simulink model "neurocircle"  (Simulink 8.3)
settings: Solver=ode3  StartTime=0.0  StopTime=1500  FixedStep=0.3  MinStep=0.01  RelTol=1e-3
libraries: simulink x3
settings Model: Creator=Administrator  LastModifiedBy=jackyjing
settings OptimizationCC: ExpressionDepthLimit=2147483647
settings DebuggingCC: FcnCallInpInsideContextMsg=UseLocalSettings

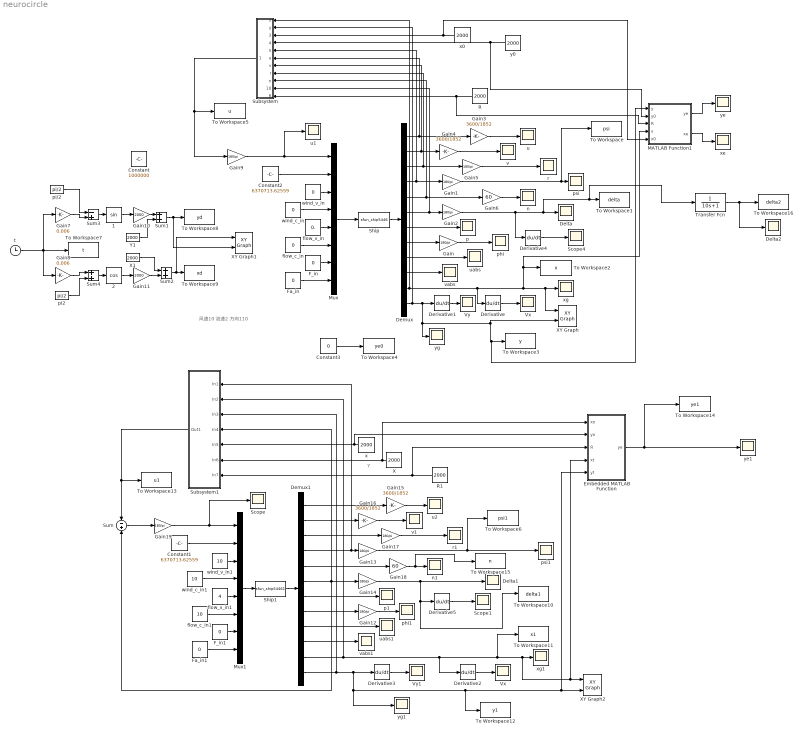
== system neurocircle ==
  note: 风速10 流速2 方向110
  note: Y
  "  1" : Trigonometry
  " 2" : Trigonometry  Operator=cos
  Constant : Constant  Value=1000000
  Constant1 : Constant  Value=6370713.62559
  Constant2 : Constant  Value=6370713.62559
  Constant3 : Constant  Value=0
  Delta : Scope
      settings: TickLabels=on  TimeRange=1500  YMin=-20  YMax=17.5  SaveName=ScopeData5
  Delta1 : Scope
      settings: TickLabels=on  TimeRange=1500  YMin=-17.5  YMax=20  SaveName=ScopeData31
  Delta2 : Scope
      settings: TickLabels=on  TimeRange=1500  YMin=-22.5  YMax=22.5  SaveName=ScopeData48
  Demux : Demux  Outputs=12
  Demux1 : Demux  Outputs=12
  Derivative{,1..5} (6 alike) : Derivative
  Embedded MATLAB Function : MATLAB Function  TreatAsAtomicUnit=on
  F_in : Constant  Value=0
  F_in1 : Constant  Value=0
  Fa_in : Constant  Value=0
  Fa_in1 : Constant  Value=0
  Gain{,1..2,5,9,12..14,17,19} (10 alike) : Gain  Gain=180/pi
  Gain10 : Gain  Gain=2000
  Gain11 : Gain  Gain=2000
  Gain{3..4,15..16} (4 alike) : Gain  Gain=3600/1852
  Gain18 : Gain  Gain=60
  Gain6 : Gain  Gain=60
  Gain7 : Gain  Gain=0.006
  Gain8 : Gain  Gain=0.006
  MATLAB Function1 : MATLAB Function  TreatAsAtomicUnit=on
  Mux : Mux  Inputs=8
  Mux1 : Mux  Inputs=8
  R : Constant  Value=2000
  R1 : Constant  Value=2000
  Scope : Scope
      settings: TimeRange=1000  YMin=-0.6  YMax=0.8  SaveName=ScopeData32
  Scope1 : Scope
      settings: YMin=-0.005  YMax=0.002  SaveName=ScopeData33
  Scope4 : Scope
      settings: YMin=-0.005  YMax=0.002  SaveName=ScopeData18
  Ship : S-Function  FunctionName=sfun_ship5446  EnableBusSupport=off
  Ship1 : S-Function  FunctionName=sfun_ship54461  EnableBusSupport=off
  Subsystem : Subsystem
  Subsystem1 : Subsystem
  Sum : Sum  Inputs=-|+
  Sum1 : Sum
  Sum2 : Sum
  Sum3 : Sum  Inputs=-+
  Sum4 : Sum
  To Workspace : ToWorkspace  VariableName=psi  SampleTime=-1
  To Workspace1 : ToWorkspace  VariableName=delta  SampleTime=-1
  To Workspace10 : ToWorkspace  VariableName=delta1  SampleTime=-1
  To Workspace11 : ToWorkspace  VariableName=x1  SampleTime=-1
  To Workspace12 : ToWorkspace  VariableName=y1  SampleTime=-1
  To Workspace13 : ToWorkspace  VariableName=u1  SampleTime=-1
  To Workspace14 : ToWorkspace  VariableName=ye1  SampleTime=-1
  To Workspace15 : ToWorkspace  VariableName=n  SampleTime=-1
  To Workspace16 : ToWorkspace  VariableName=delta2  SampleTime=-1
  To Workspace2 : ToWorkspace  VariableName=x  SampleTime=-1
  To Workspace3 : ToWorkspace  VariableName=y  SampleTime=-1
  To Workspace4 : ToWorkspace  VariableName=ye0  SampleTime=-1
  To Workspace5 : ToWorkspace  VariableName=u  SampleTime=-1
  To Workspace6 : ToWorkspace  VariableName=psi1  SampleTime=-1
  To Workspace7 : ToWorkspace  VariableName=t  SampleTime=-1
  To Workspace8 : ToWorkspace  VariableName=yd  SampleTime=-1
  To Workspace9 : ToWorkspace  VariableName=xd  SampleTime=-1
  Transfer Fcn : TransferFcn  Denominator=[10 1]
  Vx : Scope
      settings: TickLabels=on  SaveName=ScopeData8
  "Vx " : Scope
      settings: TickLabels=on  SaveName=ScopeData34
  Vy : Scope
      settings: TickLabels=on  SaveName=ScopeData9
  Vy1 : Scope
      settings: TickLabels=on  SaveName=ScopeData35
  X : Constant  Value=2000
  X1 : Constant  Value=2000
  XY Graph : simulink/Sinks/XY Graph  xmin=-1000  xmax=5000  ymin=-1000  ymax=5000  st=-1
  XY Graph1 : simulink/Sinks/XY Graph  xmin=-1000  xmax=5000  ymin=-1000  ymax=5000  st=-1
  XY Graph2 : simulink/Sinks/XY Graph  xmin=-1500  xmax=5000  ymin=-1500  ymax=5000  st=-1
  Y1 : Constant  Value=2000
  flow_c_in : Constant  Value=0
  flow_c_in1 : Constant  Value=10
  flow_v_in : Constant  Value=0.
  flow_v_in1 : Constant  Value=4
  n : Scope
      settings: TickLabels=on  YMin=38.5  YMax=46.5  SaveName=ScopeData4
  n1 : Scope
      settings: TickLabels=on  YMin=38.5  YMax=46.5  SaveName=ScopeData36
  p : Scope
      settings: TickLabels=on  SaveName=ScopeData10
  p1 : Scope
      settings: TickLabels=on  SaveName=ScopeData37
  phi : Scope
      settings: YMin=-0.00175  YMax=0.0015  SaveName=ScopeData11
  phi1 : Scope
      settings: YMin=-0.00175  YMax=0.0015  SaveName=ScopeData38
  pi/2 : Constant  Value=pi/2
  "pi2   " : Constant  Value=pi/2
  psi : Scope
      settings: TickLabels=on  TimeRange=44.44444444444434  YMin=52  YMax=60.5  SaveName=ScopeData3
  psi1 : Scope
      settings: TickLabels=on  TimeRange=500  YMin=9.9825  YMax=10.01  SaveName=ScopeData39
  r : Scope
      settings: TickLabels=on  SaveName=ScopeData2
  r1 : Scope
      settings: TickLabels=on  SaveName=ScopeData40
  t : Clock
  u : Scope
      settings: TickLabels=on  YMin=28.45  YMax=29.45
  u1 : Scope
      settings: TickLabels=on  TimeRange=1500  YMin=-35000  YMax=35000  SaveName=ScopeData15
  u2 : Scope
      settings: TickLabels=on  TimeRange=1500  YMin=10  YMax=30  SaveName=ScopeData41
  uabs : Scope
      settings: TickLabels=on  YMin=10.75  YMax=15  SaveName=ScopeData6
  uabs1 : Scope
      settings: TickLabels=on  YMin=10.75  YMax=15  SaveName=ScopeData42
  v : Scope
      settings: TickLabels=on
  v1 : Scope
      settings: TickLabels=on  YMin=-0.3  YMax=0.15  SaveName=ScopeData43
  vabs : Scope
      settings: TickLabels=on  YMin=-1.75  YMax=0  SaveName=ScopeData7
  vabs1 : Scope
      settings: TickLabels=on  YMin=-1.75  YMax=0  SaveName=ScopeData44
  wind_c_in : Constant  Value=0
  wind_c_in1 : Constant  Value=10
  wind_v_in : Constant  Value=0
  wind_v_in1 : Constant  Value=10
  x : Constant  Value=2000
  x0 : Constant  Value=2000
  xe : Scope
      settings: TickLabels=on  YMin=-475  YMax=50  SaveName=ScopeData16
  xg : Scope
      settings: TickLabels=on  YMin=250  YMax=475  SaveName=ScopeData12
  xg1 : Scope
      settings: TickLabels=on  YMin=-100  YMax=1100  SaveName=ScopeData45
  y0 : Constant  Value=2000
  ye : Scope
      settings: TickLabels=on  YMin=-550  YMax=250  SaveName=ScopeData17
  ye1 : Scope
      settings: TickLabels=on  YMin=-100  YMax=850  SaveName=ScopeData47
  yg : Scope
      settings: TickLabels=on  YMin=250  YMax=475  SaveName=ScopeData13
  yg1 : Scope
      settings: TickLabels=on  YMin=-800  YMax=600  SaveName=ScopeData46
  wires:
  Ship/1 -> Demux/1
  Demux/1 -> Subsystem/6(u), Gain3/1
  Demux/2 -> Subsystem/7(v), Gain4/1
  Demux/3 -> Subsystem/8(r), Gain5/1
  Demux/5 -> Subsystem/9(n), Gain6/1
  Demux/7 -> p/1
  Demux/8 -> Gain/1
  Demux/4 -> Gain1/1, Subsystem/5(psi)
  Gain/1 -> phi/1
  Gain3/1 -> u/1
  Gain4/1 -> v/1
  Gain5/1 -> r/1
  Gain6/1 -> n/1
  Demux/9 -> uabs/1
  Demux/10 -> vabs/1
  Demux/12 -> Subsystem/2(y), Derivative1/1, yg/1, MATLAB Function1/1(y), To Workspace3/1, XY Graph/2
  Demux/11 -> Subsystem/1(x), Derivative/1, XY Graph/1, xg/1, MATLAB Function1/4(x), To Workspace2/1
  Derivative/1 -> Vx/1
  Derivative1/1 -> Vy/1
  wind_v_in/1 -> Mux/3
  wind_c_in/1 -> Mux/4
  flow_v_in/1 -> Mux/5
  F_in/1 -> Mux/7
  Fa_in/1 -> Mux/8
  flow_c_in/1 -> Mux/6
  Mux/1 -> Ship/1
  Constant2/1 -> Mux/2
  Derivative4/1 -> Scope4/1
  Gain9/1 -> u1/1, Mux/1
  y0/1 -> MATLAB Function1/2(y0), Subsystem/4(y0)
  R/1 -> MATLAB Function1/3(R), Subsystem/11(R)
  Sum1/1 -> XY Graph1/2, To Workspace8/1
  "  1"/1 -> Gain10/1
  " 2"/1 -> Gain11/1
  t/1 -> To Workspace7/1, Gain8/1, Gain7/1
  Gain10/1 -> Sum1/1
  Gain11/1 -> Sum2/2
  X1/1 -> Sum2/1
  Y1/1 -> Sum1/2
  Sum3/1 -> "  1"/1
  Gain7/1 -> Sum3/2
  pi/2/1 -> Sum3/1
  Sum4/1 -> " 2"/1
  Gain8/1 -> Sum4/1
  "pi2   "/1 -> Sum4/2
  Demux/6 -> Subsystem/10(Delta), Gain2/1
  Subsystem/1("psi ") -> To Workspace5/1, Gain9/1
  MATLAB Function1/2(xe) -> xe/1
  MATLAB Function1/1(ye) -> ye/1
  x0/1 -> MATLAB Function1/5(x0), Subsystem/3(x0)
  Gain1/1 -> psi/1, To Workspace/1
  Sum2/1 -> XY Graph1/1, To Workspace9/1
  Ship1/1 -> Demux1/1
  Demux1/1 -> Gain15/1
  Demux1/2 -> Gain16/1
  Demux1/3 -> Gain17/1
  Demux1/5 -> Gain18/1
  Demux1/7 -> p1/1
  Demux1/8 -> Gain12/1
  Gain13/1 -> psi1/1, To Workspace6/1
  Gain12/1 -> phi1/1
  Gain15/1 -> u2/1
  Gain16/1 -> v1/1
  Gain17/1 -> r1/1
  Gain18/1 -> To Workspace15/1, n1/1
  Demux1/9 -> uabs1/1
  Demux1/10 -> vabs1/1
  Demux1/12 -> Derivative3/1, yg1/1, To Workspace12/1, Embedded MATLAB Function/5(yt), XY Graph2/2, Subsystem1/3(In3)
  Demux1/11 -> Derivative2/1, To Workspace11/1, Embedded MATLAB Function/4(xt), XY Graph2/1, xg1/1, Subsystem1/2(In2)
  Derivative2/1 -> "Vx "/1
  Derivative3/1 -> Vy1/1
  wind_v_in1/1 -> Mux1/3
  wind_c_in1/1 -> Mux1/4
  flow_v_in1/1 -> Mux1/5
  F_in1/1 -> Mux1/7
  Fa_in1/1 -> Mux1/8
  flow_c_in1/1 -> Mux1/6
  Mux1/1 -> Ship1/1
  Constant1/1 -> Mux1/2
  Sum/1 -> Gain19/1
  Derivative5/1 -> Scope1/1
  Subsystem1/1(Out1) -> Sum/1, To Workspace13/1
  Demux1/4 -> Gain13/1, Subsystem1/1(In1)
  Gain19/1 -> Mux1/1, Scope/1
  x/1 -> Subsystem1/5(In5), Embedded MATLAB Function/2(yo)
  X/1 -> Subsystem1/6(In6), Embedded MATLAB Function/1(xo)
  R1/1 -> Subsystem1/7(In7), Embedded MATLAB Function/3(R)
  Demux1/6 -> Sum/2, Gain14/1, Subsystem1/4(In4)
  Gain14/1 -> To Workspace10/1, Derivative5/1, Delta1/1
  Embedded MATLAB Function/1(ye) -> ye1/1, To Workspace14/1
  Constant3/1 -> To Workspace4/1
  Gain2/1 -> Derivative4/1, Delta/1, Transfer Fcn/1, To Workspace1/1
  Transfer Fcn/1 -> Delta2/1, To Workspace16/1

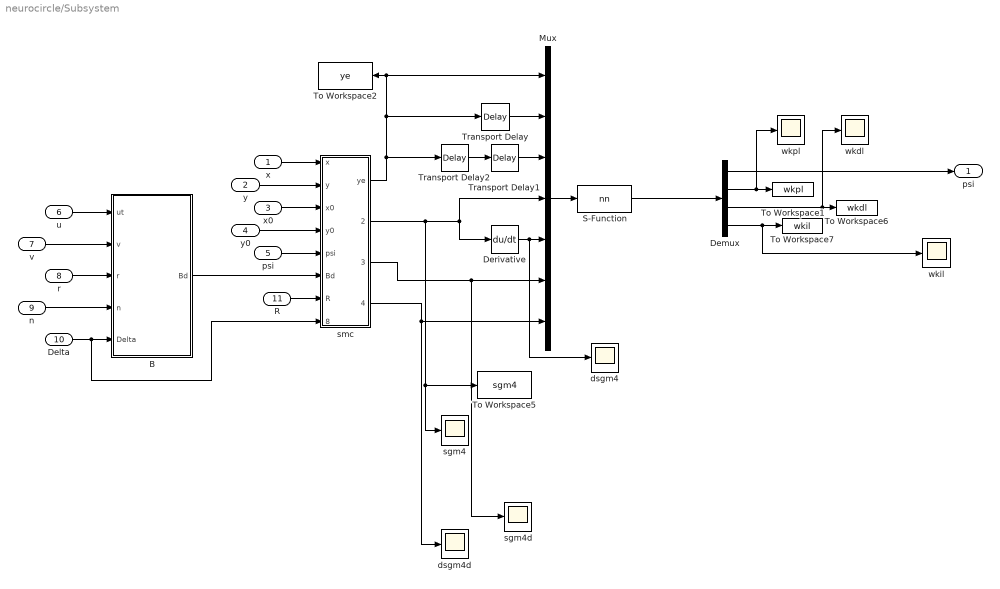
== system neurocircle/Subsystem ==
  x : Inport
  y : Inport  Port=2
  x0 : Inport  Port=3
  y0 : Inport  Port=4
  psi : Inport  Port=5
  u : Inport  Port=6
  v : Inport  Port=7
  r : Inport  Port=8
  n : Inport  Port=9
  Delta : Inport  Port=10
  R : Inport  Port=11
  B : MATLAB Function  TreatAsAtomicUnit=on
  Demux : Demux
  Derivative : Derivative
  Mux : Mux  Inputs=7
  S-Function : S-Function  FunctionName=nn  EnableBusSupport=off
  To Workspace1 : ToWorkspace  VariableName=wkpl  SampleTime=-1
  To Workspace2 : ToWorkspace  VariableName=ye  SampleTime=-1
  To Workspace5 : ToWorkspace  VariableName=sgm4  SampleTime=-1
  To Workspace6 : ToWorkspace  VariableName=wkdl  SampleTime=-1
  To Workspace7 : ToWorkspace  VariableName=wkil  SampleTime=-1
  Transport Delay : TransportDelay  DelayTime=2
  Transport Delay1 : TransportDelay
  Transport Delay2 : TransportDelay
  dsgm4 : Scope
      settings: TickLabels=on  TimeRange=1500  YMin=-4.20046e+11  YMax=-3.80042e+11  SaveName=ScopeData25
  dsgm4d : Scope
      settings: TickLabels=on  TimeRange=1500  YMin=0.00019  YMax=0.00028  SaveName=ScopeData23
  sgm4 : Scope
      settings: TickLabels=on  TimeRange=1500  YMin=-0.00045  YMax=0.0006  SaveName=ScopeData24
  sgm4d : Scope
      settings: TickLabels=on  TimeRange=1500  YMin=0.00975  YMax=0.014  SaveName=ScopeData21
  "smc " : Subsystem
  wkdl : Scope
      settings: TickLabels=on  TimeRange=1500  YMin=0.3  YMax=1  SaveName=ScopeData19
  wkil : Scope
      settings: TickLabels=on  TimeRange=1500  YMin=-0.025  YMax=0.35  SaveName=ScopeData20
  wkpl : Scope
      settings: TickLabels=on  TimeRange=1500  YMin=-0.45  YMax=0.5  SaveName=ScopeData22
  "psi " : Outport
  wires:
  x/1 -> "smc "/1(x)
  y/1 -> "smc "/2(y)
  x0/1 -> "smc "/3(x0)
  y0/1 -> "smc "/4(y0)
  psi/1 -> "smc "/5("psi ")
  u/1 -> B/1(ut)
  v/1 -> B/2(v)
  r/1 -> B/3(r)
  n/1 -> B/4(n)
  Mux/1 -> S-Function/1
  Transport Delay/1 -> Mux/2
  Transport Delay1/1 -> Mux/3
  Derivative/1 -> dsgm4/1, Mux/5
  B/1(Bd) -> "smc "/6(Bd)
  Transport Delay2/1 -> Transport Delay1/1
  R/1 -> "smc "/7(R)
  Delta/1 -> "smc "/8(delta), B/5(Delta)
  S-Function/1 -> Demux/1
  Demux/2 -> To Workspace1/1, wkpl/1
  Demux/3 -> To Workspace6/1, wkdl/1
  Demux/4 -> wkil/1, To Workspace7/1
  Demux/1 -> "psi "/1
  "smc "/1(ye) -> Transport Delay2/1, Transport Delay/1, Mux/1, To Workspace2/1
  "smc "/2(sgm4) -> Mux/4, Derivative/1, To Workspace5/1, sgm4/1
  "smc "/3(sgm4d) -> sgm4d/1, Mux/6
  "smc "/4(dsgm4d) -> Mux/7, dsgm4d/1

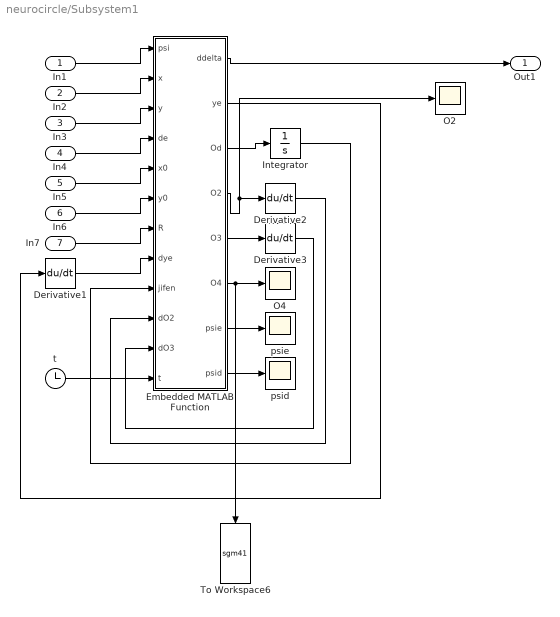
== system neurocircle/Subsystem1 ==
  In1 : Inport
  In2 : Inport  Port=2
  In3 : Inport  Port=3
  In4 : Inport  Port=4
  In5 : Inport  Port=5
  In6 : Inport  Port=6
  In7 : Inport  Port=7
  Derivative1 : Derivative
  Derivative2 : Derivative
  Derivative3 : Derivative
  Embedded MATLAB Function : MATLAB Function  TreatAsAtomicUnit=on
  Integrator : Integrator
  O2 : Scope
      settings: TickLabels=on  TimeRange=500  YMin=-4.5  YMax=3.5  SaveName=ScopeData19
  O4 : Scope
      settings: TickLabels=on  TimeRange=500  YMin=-0.00115  YMax=-0.0001  SaveName=ScopeData18
  To Workspace6 : ToWorkspace  VariableName=sgm41  SampleTime=-1
  psid : Scope
      settings: TickLabels=on  TimeRange=2000  YMin=-2  SaveName=ScopeData20
  psie : Scope
      settings: TickLabels=on  TimeRange=2000  YMin=0.1  YMax=0.8  SaveName=ScopeData17
  t : Clock
  Out1 : Outport
  wires:
  Embedded MATLAB Function/5(O3) -> Derivative3/1
  Derivative3/1 -> Embedded MATLAB Function/11(dO3)
  Embedded MATLAB Function/4(O2) -> O2/1, Derivative2/1
  Derivative2/1 -> Embedded MATLAB Function/10(dO2)
  Integrator/1 -> Embedded MATLAB Function/9(jifen)
  Embedded MATLAB Function/1(ddelta) -> Out1/1
  Embedded MATLAB Function/3(Od) -> Integrator/1
  In1/1 -> Embedded MATLAB Function/1(psi)
  In2/1 -> Embedded MATLAB Function/2(x)
  In3/1 -> Embedded MATLAB Function/3(y)
  Derivative1/1 -> Embedded MATLAB Function/8(dye)
  Embedded MATLAB Function/2(ye) -> Derivative1/1
  In4/1 -> Embedded MATLAB Function/4(de)
  In5/1 -> Embedded MATLAB Function/5(x0)
  In6/1 -> Embedded MATLAB Function/6(y0)
  In7/1 -> Embedded MATLAB Function/7(R)
  Embedded MATLAB Function/7(psie) -> psie/1
  Embedded MATLAB Function/6(O4) -> O4/1, To Workspace6/1
  Embedded MATLAB Function/8(psid) -> psid/1
  t/1 -> Embedded MATLAB Function/12(t)

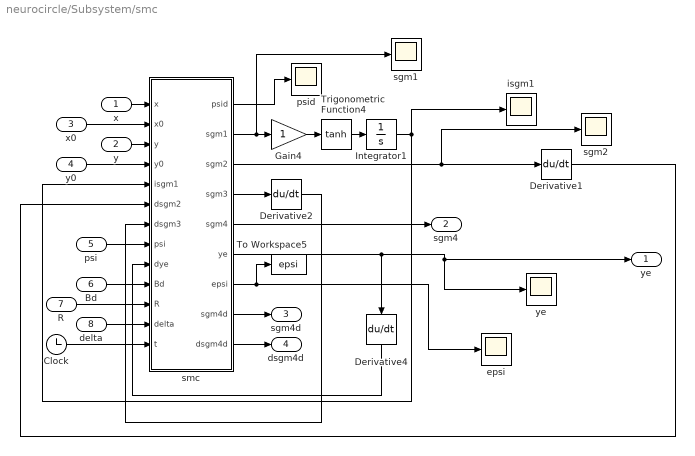
== system neurocircle/Subsystem/smc  ==
  x : Inport
  y : Inport  Port=2
  x0 : Inport  Port=3
  y0 : Inport  Port=4
  "psi " : Inport  Port=5
  Bd : Inport  Port=6
  R : Inport  Port=7
  delta : Inport  Port=8
  Clock : Clock
  Derivative1 : Derivative
  Derivative2 : Derivative
  Derivative4 : Derivative
  Gain4 : Gain
  Integrator1 : Integrator
  To Workspace5 : ToWorkspace  VariableName=epsi  SampleTime=-1
  Trigonometric Function4 : Trigonometry  Operator=tanh
  epsi : Scope
      settings: TickLabels=on  TimeRange=1500  YMin=-0.1  YMax=0.8  SaveName=ScopeData29
  isgm1 : Scope
      settings: TickLabels=on  TimeRange=1500  YMin=-150  YMax=650  SaveName=ScopeData28
  psid : Scope
      settings: TickLabels=on  TimeRange=1500  YMin=-3.5  YMax=3.5  SaveName=ScopeData30
  sgm1 : Scope
      settings: TickLabels=on  TimeRange=1500  YMin=-15  YMax=15  SaveName=ScopeData26
  sgm2 : Scope
      settings: TickLabels=on  TimeRange=1500  YMax=7  SaveName=ScopeData27
  "smc " : MATLAB Function  TreatAsAtomicUnit=on
  "ye " : Scope
      settings: TimeRange=1500  YMin=-700  YMax=900  SaveName=ScopeData14
  ye : Outport
  sgm4 : Outport  Port=2
  sgm4d : Outport  Port=3
  dsgm4d : Outport  Port=4
  wires:
  "smc "/2(sgm1) -> sgm1/1, Gain4/1
  Derivative2/1 -> "smc "/7(dsgm3)
  "smc "/4(sgm3) -> Derivative2/1
  Trigonometric Function4/1 -> Integrator1/1
  Derivative1/1 -> "smc "/6(dsgm2)
  Integrator1/1 -> isgm1/1, "smc "/5(isgm1)
  x/1 -> "smc "/1(x)
  y/1 -> "smc "/3(y)
  x0/1 -> "smc "/2(x0)
  y0/1 -> "smc "/4(y0)
  "smc "/5(sgm4) -> sgm4/1
  "smc "/6(ye) -> "ye "/1, ye/1, Derivative4/1
  Bd/1 -> "smc "/10(Bd)
  Derivative4/1 -> "smc "/9(dye)
  "smc "/8(sgm4d) -> sgm4d/1
  "smc "/9(dsgm4d) -> dsgm4d/1
  R/1 -> "smc "/11(R)
  delta/1 -> "smc "/12(delta)
  "smc "/7(epsi) -> To Workspace5/1, epsi/1
  Gain4/1 -> Trigonometric Function4/1
  "smc "/1(psid) -> psid/1
  "psi "/1 -> "smc "/8(psi)
  "smc "/3(sgm2) -> Derivative1/1, sgm2/1
  Clock/1 -> "smc "/13(t)

== matlab function Subsystem/smc /smc  ==
  data: psid output double; x input double; x0 input double; y input double; y0 input double; isgm1 input double; dsgm2 input double; dsgm3 input double; sgm1 output double; sgm2 output double; sgm3 output double; psi input double; dye input double; sgm4 output double; ye output double; epsi output double; Bd input double; sgm4d output double; dsgm4d output double; R input double; delta input double; t input double
function [psid,sgm1,sgm2,sgm3,sgm4,ye,epsi,sgm4d,dsgm4d]= fcn(x,x0,y,y0,isgm1,dsgm2,dsgm3,psi,dye,Bd,R,delta,t)
%#codegen
% k0=0.8;k1=3;k2=0.0000001;k3=0.0000002;k4=0.04;
%k0=0.8;k1=0.001;k2=0.0000001;k3=0.0000002;k4=0.04;
k0=0.8;k1=4;k2=0.0000001;k3=0.0000001;k4=0.03;
 ye=sqrt((x-x0)^2+(y-y0)^2)-R;
if(atan2((y-y0),(x-x0))<0&&t>700)
    epsi=psi-atan2((y-y0),(x-x0))-pi/2-2*pi;
elseif(atan2((y-y0),(x-x0))>0&&t>1000)
    epsi=psi-atan2((y-y0),(x-x0))-pi/2-2*pi;
else
    epsi=psi-atan2((y-y0),(x-x0))-pi/2;     
end

  psid=atan2((y-y0),(x-x0));
% if(t<=784.2)
%   epsi=psi-psid-pi/2;
% else
%   epsi=0.0473;
% end
% epsi=psi-psid-pi/2;
sgm1=k1*tanh(k0*ye)+dye;
sgm2=epsi+k2*isgm1;
sgm3=k3*tanh(sgm2)+dsgm2;
sgm4=k4*tanh(sgm3)+dsgm3;

sgm4d=Bd; 
dsgm4d=(k4*(sech(sgm3)^2)+k3*(sech(sgm2)^2))*Bd;

== matlab function Subsystem/B ==
  data: ut input double; Bd output double; v input double; r input double; n input double; Delta input double
function Bd  = fcn(ut,v,r,n,Delta)
% function ud = fcn(ut,v,r,n,Delta,phi,dr,sgm4)
V=sqrt(ut*ut+v*v);%u=x(1) v=x(2)

da=10.5;%9.34+0.25;%尾吃水13.8;%12.5;%
df=7.5;%4.97+0.25;%首吃水14.3;%13.8;%
Dh=9.0;%舵高s   ;%11.411.4;;%+7.00+0.25
pa=1.205;%%%**空气密度
Lpp=267.0;%船长
B=39.8;%船宽
Db=6.466;%舵宽
P=9.657;%da螺距
luow=1026;%小luow是密度 水密度
Dp=9.2;%螺旋桨直径
Ds=23.6;%型深
d=(da+df)/2;%吃水
m=(165.89*d*d + 4383.9*d)*1000;%排水量
Cb=m/(Lpp*B*d*1.025*1000);
AR=(d-7.41)/(12.5-7.41)*(81.44-43.14)+43.14;%舵叶面积
d_B=d/B;L_B=Lpp/B;
mx=m/100*(0.398+11.97*Cb*(1+3.73*d_B)-2.89*Cb*L_B*(1+1.13*d_B)+0.175*Cb*L_B*L_B*(1+0.541*d_B)-1.107*L_B*d_B);
my=m*(0.882-0.54*Cb*(1-1.6*d_B)-0.156*L_B*(1-0.673*Cb)+0.826*d_B*L_B*(1-0.678*d_B)-0.638*Cb*d_B*L_B*(1-0.669*d_B));
wp0=0.5*Cb-0.05;
fa=6.13*Dh/Db/(2.25+Dh/Db);
gma=-22.2*(Cb*B/Lpp)*(Cb*B/Lpp)+0.02*(Cb*B/Lpp)+0.68;
gmaR=1.1633-1.98828*Cb+1.3902*Cb*Cb;
tR=0.7382-0.0539*Cb+0.1755*Cb*Cb;
ifaH=0.6784-1.3374*Cb+1.8891*Cb*Cb;
xH=-(0.4+0.1*Cb)*Lpp;
xR=-0.5*Lpp;
xb=1.87;
Jzz=1/100.0*(33-76.85*Cb*(1-0.784*Cb)+3.43*L_B*(1-0.63*Cb))*Lpp*Lpp;
Izz=(1.0+(Cb^4.5))*m*(Lpp*Lpp+power(B,2.4))/24.0;

m33=Izz+Jzz;

beta=atan2((-v),(ut));%u=x(1) v=x(2)
betap=beta+0.5*r*Lpp/V;%r=x(3)
betaR=beta+r*Lpp/V;
wp=wp0*exp(-4.0*betap*betap);
up=(1.0-wp)*ut;%u=x(1)
s=1.0-up/n/P;% n=x(5)
eta=Dp/Dh;

k=0.6;
Gs=eta*k*(2.0-(2.0-k)*s)*s/(1.0-s)/(1.0-s);
s0=1-(1-wp0)*ut/n/P;% n=x(5)u=x(1)
delt0=-s0/57.3;

if(Delta<0)
    K=1.065;
else
    K=0.935;
end
%
uR=up*(1+K*Gs)^0.5;
vRp=uR*delt0;
vR=vRp-gmaR*(v-Lpp*r);%r=x(3)v=x(2)
UR2=uR*uR+vR*vR;
J=ut*(1-wp)/n/Dp;%u=x(1)  n=x(5)
if(J<=0.3)
    L_ifaH=ifaH*J/0.3;% p137, 3-5-119
else
    L_ifaH=ifaH;
end
%
Bd=(-1.0/2.0)*(xR+L_ifaH*xH)*luow*AR*fa*UR2*cos(Delta)/(m33);

== matlab function Embedded MATLAB Function ==
  data: xo input double; yo input double; R input double; xt input double; ye output double; yt input double
function ye = fcn(xo,yo,R,xt,yt)
%#eml
ye=(sqrt((xo-xt)^2+(yo-yt)^2)-R);

== matlab function MATLAB Function1 ==
  data: y input double; ye output double; y0 input double; R input double; x input double; x0 input double; xe output double
function [ye,xe]= fcn(y,y0,R,x,x0)
%#codegen

thta=atan2((y-y0),(x-x0));
xe = x-x0-R*cos(thta);
ye = y-y0-R*sin(thta);

== matlab function Subsystem1/Embedded MATLAB Function ==
  data: psi input double; x input double; y input double; de input double; x0 input double; y0 input double; R input double; dye input double; ddelta output double; ye output double; Od output double; O2 output double; O3 output double; O4 output double; jifen input double; dO2 input double; dO3 input double; psie output double; psid output double; t input double
function [ddelta,ye,Od,O2,O3,O4,psie,psid] = fcn(psi,x,y,de,x0,y0,R,dye,jifen,dO2,dO3,t)
K0=0.01;K1=2;K2=0.05;K3=0.005;K4=0.01;
K5=5;Te=2.5;

ye=sqrt((x-x0)^2+(y-y0)^2)-R;
% if(de>0)
%     psie=psi-atan2((y-y0),(x-x0))-pi/2;
% else
%     psie=psi-atan2((y-y0),(x-x0))+pi/2;
% end
psid=atan2((y-y0),(x-x0))+pi/2;
%psie=psi-atan2((y-y0),(x-x0))-pi/2;
if(atan2((y-y0),(x-x0))<0&&t>700)
    psie=psi-atan2((y-y0),(x-x0))-pi/2-2*pi;
elseif(atan2((y-y0),(x-x0))>0&&t>1000)
    psie=psi-atan2((y-y0),(x-x0))-pi/2-2*pi;
else
    psie=psi-atan2((y-y0),(x-x0))-pi/2;     
end
O1=K1*f(K0*ye)+dye;
Od=f(O1);
O2=psie+K2*jifen;
O3=K3*f(O2)+dO2;
O4=K4*f(O3)+dO3;
ddelta=-Te*K5*O4;
 function mean=f(a)
  mean=tanh(a);
%  function mean=f(a)
%  if(a<0.1&&a>-0.1)
%      mean=a;
%  else
%      mean=coth(a)-1/a;
%  end
